simulink model "elevator_alt"  (R2014a)
settings: Solver=ode45  StartTime=0.0  StopTime=100000000  RelTol=1e-3
settings Model: Creator=Rishabh  LastModifiedBy=Rishabh

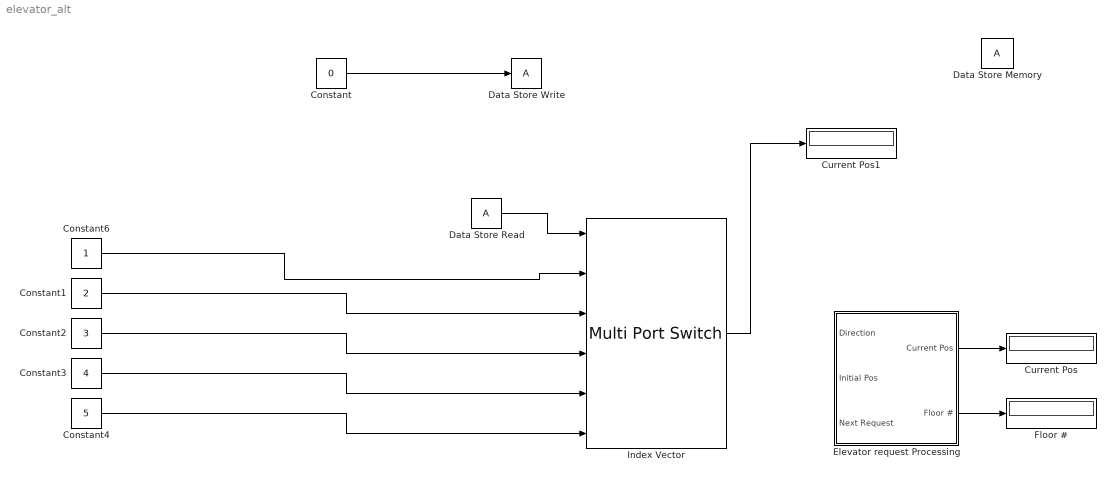
== system elevator_alt ==
  Constant : Constant  Value=0
  Constant1 : Constant  Value=2
  Constant2 : Constant  Value=3
  Constant3 : Constant  Value=4
  Constant4 : Constant  Value=5
  Constant6 : Constant
  Current Pos : Display
  Current Pos1 : Display
  Data Store Memory : DataStoreMemory  ReadBeforeWriteMsg=warning  WriteAfterWriteMsg=warning  WriteAfterReadMsg=warning
  Data Store Read : DataStoreRead
  Data Store Write : DataStoreWrite
  Elevator request Processing : Subsystem
  Floor # : Display
  Index Vector : MultiPortSwitch  DataPortOrder=Zero-based contiguous  Inputs=5  zeroidx=on
  wires:
  Constant4/1 -> Index Vector/6
  Constant3/1 -> Index Vector/5
  Constant2/1 -> Index Vector/4
  Constant1/1 -> Index Vector/3
  Constant6/1 -> Index Vector/2
  Data Store Read/1 -> Index Vector/1
  Constant/1 -> Data Store Write/1
  Index Vector/1 -> Current Pos1/1
  Elevator request Processing/2(Floor #) -> Floor #/1
  Elevator request Processing/1(Current Pos) -> Current Pos/1

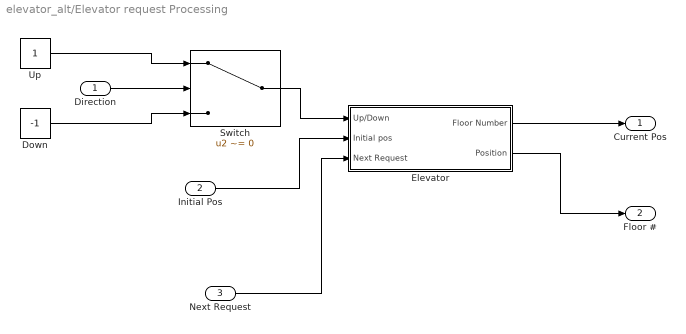
== system elevator_alt/Elevator request Processing ==
  Direction : Inport
  Initial Pos : Inport  Port=2
  Next Request : Inport  Port=3
  Down : Constant  Value=-1
  Elevator : Subsystem
  Switch : Switch  Criteria=u2 ~= 0
  Up : Constant
  Current Pos : Outport
  Floor # : Outport  Port=2
  wires:
  Up/1 -> Switch/1
  Direction/1 -> Switch/2
  Switch/1 -> Elevator/1(Up/Down)
  Down/1 -> Switch/3
  Next Request/1 -> Elevator/3(Next Request)
  Elevator/1(Floor Number) -> Current Pos/1
  Elevator/2(Position) -> Floor #/1
  Initial Pos/1 -> Elevator/2(Initial pos)

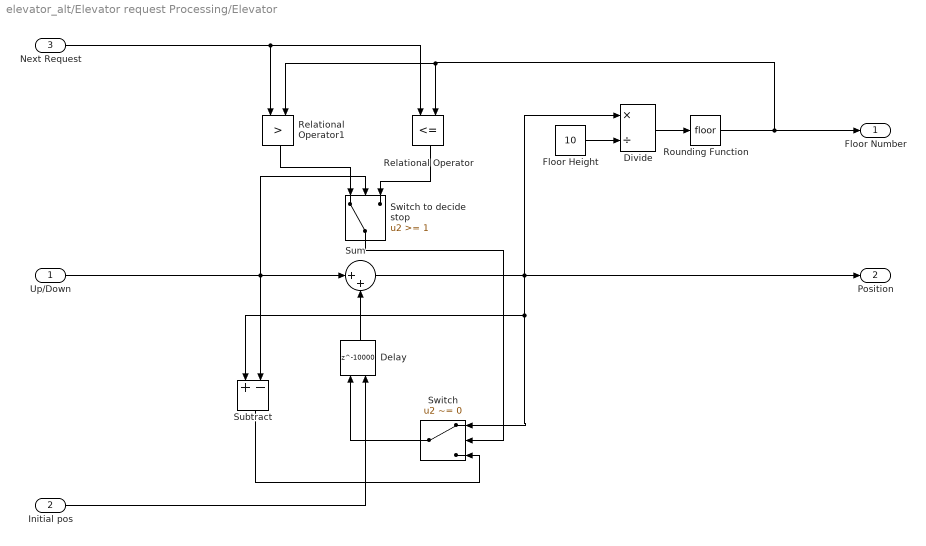
== system elevator_alt/Elevator request Processing/Elevator ==
  Up/Down : Inport
  Initial pos : Inport  Port=2
  Next Request : Inport  Port=3
  Delay : Delay  DelayLength=10000  InitialConditionSource=Input port  InitialCondition=2  SampleTime=.00001
      settings: InputPortMap=u0,p4
  Divide : Product  Inputs=*/  RndMeth=Nearest  LockScale=on
  Floor Height : Constant  Value=10
  Relational Operator : RelationalOperator  Operator=<=  OutDataTypeStr=boolean
  Relational Operator1 : RelationalOperator  Operator=>  OutDataTypeStr=boolean
  Rounding Function : Rounding
  Subtract : Sum  Inputs=+-
  Sum : Sum  Inputs=|++
  Switch : Switch  Criteria=u2 ~= 0
  Switch to decide stop : Switch  Threshold=1
  Floor Number : Outport
  Position : Outport  Port=2
  wires:
  Delay/1 -> Sum/2
  Up/Down/1 -> Switch to decide stop/2, Sum/1, Subtract/2
  Sum/1 -> Position/1, Subtract/1, Switch/1, Divide/1
  Divide/1 -> Rounding Function/1
  Floor Height/1 -> Divide/2
  Rounding Function/1 -> Relational Operator1/2, Relational Operator/2, Floor Number/1
  Relational Operator/1 -> Switch to decide stop/3
  Next Request/1 -> Relational Operator1/1, Relational Operator/1
  Switch/1 -> Delay/1
  Relational Operator1/1 -> Switch to decide stop/1
  Switch to decide stop/1 -> Switch/2
  Subtract/1 -> Switch/3
  Initial pos/1 -> Delay/2
